simulink model "Function3_2018a"  (R2018a)
settings: Solver=FixedStepDiscrete  StartTime=0.0  StopTime=0.1  FixedStep=0.1  RelTol=1e-3  EnableMultiTasking=on
settings Model: Creator=bzhan  LastModifiedBy=bzhan
settings SolverCC: AutoInsertRateTranBlk=on
settings DataIOCC: LimitDataPoints=on  ReturnWorkspaceOutputs=on
settings OptimizationCC: LifeSpan=inf
settings DebuggingCC: AllowSymbolicDim=off  SFUnexpectedBacktrackingDiag=warning  SFNoUnconditionalDefaultTransitionDiag=warning  SFExecutionAtInitializationDiag=none
settings CodeAppCC: StateflowObjectComments=on
settings GRTTargetCC: TargetLangStandard=C89/C90 (ANSI)
settings ConfigComp: CovMetricSettings=dw  CovHtmlReporting=on  CovSaveCumulativeToWorkspaceVar=on  CovSaveSingleToWorkspaceVar=on  CovShowResultsExplorer=off  CovExternalEMLEnable=off  CovSFcnEnable=off

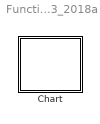
== system Function3_2018a ==
  Chart : Stateflow chart  TreatAsAtomicUnit=on

== stateflow chart Function3_2018a/Chart ==
  state A
    en: f("en_A")
  state B
    en: f("en_B")
  (default) -> A : {b=[0,1,2];}
  A -> (junction 29) : {compute()}
  (junction 29) -> B : [a(1)==0 && a(2)==2 && a(3)==4]
  data: s function_input; a local double size=1 3 =[0 0 0]; b local double size=1 3 =[0 0 0]
  function compute:
    | function compute
    |   a(1) = b(1);
    |   a(2) = b(2)+1;
    |   a(3) = b(3)+2;
  function f(s):
    | function f(s)
    |   fprintf(s+"\n");
